simulink model "Adjoint_MIMO_supp"  (R2017b)
settings: Solver=ode4  StartTime=0.0  StopTime=Tend  FixedStep=Ts  RelTol=1e-3  EnableMultiTasking=on
values from neighbouring files (symbols this model uses):
  Arc = [0 0 0 -3.79740657573 0.00492323855906 0.0757867668346 0 0 0 0 0 0 ... (144 elements, 12x12)]    [longlatParameters.mat]
  Brc = [0 0 0 0.4753435248 -0.00046 0 0 0 0 0 0 0 ... (48 elements, 12x4)]    [longlatParameters.mat]
  Crc = [1 0 0 0 0 0 1 0 0 0 0 0 ... (48 elements, 4x12)]    [longlatParameters.mat]
  flag_x = 1    [IdealTrack_v3_longlat.m]
  flag_y = 1    [IdealTrack_v3_longlat.m]
  flag_z = 1    [IdealTrack_v3_longlat.m]
settings Model: Creator=WhisPer  LastModifiedBy=Jinrui
settings DataIOCC: LimitDataPoints=on
settings OptimizationCC: LifeSpan=inf
settings DebuggingCC: AllowSymbolicDim=off  SFUnexpectedBacktrackingDiag=warning  SFNoUnconditionalDefaultTransitionDiag=warning  SFExecutionAtInitializationDiag=none
settings ModelReferenceCC: PropagateSignalLabelsOutOfModel=off
settings CodeAppCC: StateflowObjectComments=on
settings GRTTargetCC: TargetLangStandard=C89/C90 (ANSI)
settings ConfigComp: CovMetricSettings=dw  CovHtmlReporting=on  CovSaveCumulativeToWorkspaceVar=on  CovSaveSingleToWorkspaceVar=on  CovExternalEMLEnable=off

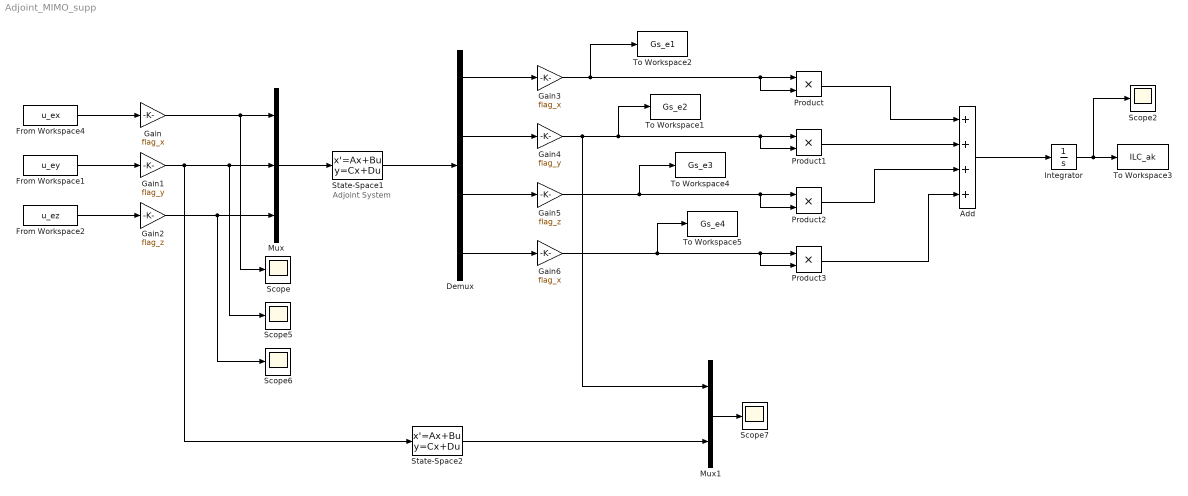
== system Adjoint_MIMO_supp ==
  note: Adjoint System
  Add : Sum  Inputs=++++
  Demux : Demux
  From Workspace1 : FromWorkspace  VariableName=u_ey  SampleTime=0
  From Workspace2 : FromWorkspace  VariableName=u_ez  SampleTime=0
  From Workspace4 : FromWorkspace  VariableName=u_ex  SampleTime=0
  Gain : Gain  Gain=flag_x
  Gain1 : Gain  Gain=flag_y
  Gain2 : Gain  Gain=flag_z
  Gain3 : Gain  Gain=flag_x
  Gain4 : Gain  Gain=flag_y
  Gain5 : Gain  Gain=flag_z
  Gain6 : Gain  Gain=flag_x
  Integrator : Integrator
  Mux : Mux  Inputs=3
  Mux1 : Mux  Inputs=2
  Product{,1..3} (4 alike) : Product
  Scope{,2,5..7} (5 alike) : Scope
  State-Space1 : StateSpace  A=Arc'  B=Crc(1:3,:)'  C=Brc'  D=zeros(4,3)  InitialCondition=0
  State-Space2 : StateSpace  A=Arc(7:12,7:12)'  B=Crc(2,7:12)'  C=Brc(7:12,2)'  D=0  InitialCondition=0
  To Workspace1 : ToWorkspace  VariableName=Gs_e2  SampleTime=-1
  To Workspace2 : ToWorkspace  VariableName=Gs_e1  SampleTime=-1
  To Workspace3 : ToWorkspace  VariableName=ILC_ak  SampleTime=-1
  To Workspace4 : ToWorkspace  VariableName=Gs_e3  SampleTime=-1
  To Workspace5 : ToWorkspace  VariableName=Gs_e4  SampleTime=-1
  wires:
  Integrator/1 -> Scope2/1, To Workspace3/1
  Demux/1 -> Gain3/1
  Demux/2 -> Gain4/1
  Demux/3 -> Gain5/1
  Product1/1 -> Add/2
  Product/1 -> Add/1
  Product2/1 -> Add/3
  Add/1 -> Integrator/1
  From Workspace4/1 -> Gain/1
  From Workspace1/1 -> Gain1/1
  From Workspace2/1 -> Gain2/1
  Gain/1 -> Scope/1, Mux/1
  Gain1/1 -> State-Space2/1, Scope5/1, Mux/2
  Gain2/1 -> Scope6/1, Mux/3
  Mux/1 -> State-Space1/1
  Gain3/1 -> To Workspace2/1, Product/2, Product/1
  State-Space2/1 -> Mux1/2
  Mux1/1 -> Scope7/1
  Product3/1 -> Add/4
  Demux/4 -> Gain6/1
  State-Space1/1 -> Demux/1
  Gain4/1 -> Mux1/1, To Workspace1/1, Product1/2, Product1/1
  Gain5/1 -> To Workspace4/1, Product2/2, Product2/1
  Gain6/1 -> To Workspace5/1, Product3/1, Product3/2
